simulink library "filteredPID_ul"  (R2022a)
settings: Solver=VariableStepAuto  StartTime=0.0  StopTime=10.0  RelTol=1e-3
settings Model: Creator=adabney  LastModifiedBy=adabney

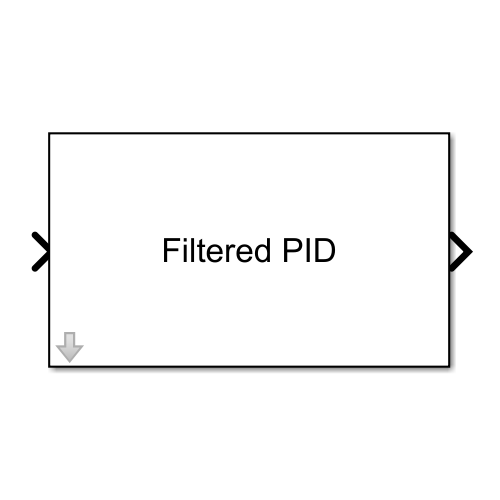
[thumbnail: Simulink's stored preview of the top-level diagram]
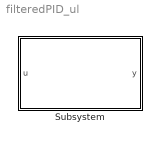
== system filteredPID_ul ==
  Subsystem : Subsystem  mask{kp=0, ki=0, kd=0, tau=0}
      mask prompts: kp "Proportional Gain"; ki "Integral Gain"; kd "Derivative Gain"; tau "Filter Time Constant"
      mask DialogControl ParameterGroupVar Prompt: Control Gains
      mask Display: disp('Filtered PID');

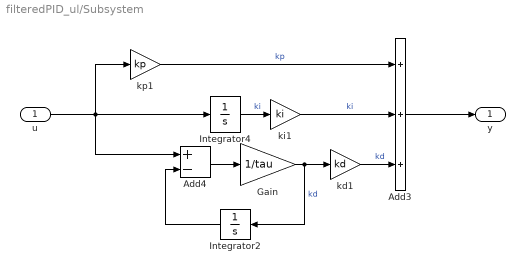
== system filteredPID_ul/Subsystem ==
  u : Inport  PortDimensions=1
  Add3 : Sum  Inputs=+++
  Add4 : Sum  Inputs=+-
  Gain : Gain  Gain=1/tau
  Integrator2 : Integrator  ContinuousStateAttributes='ctrlDerivative'
  Integrator4 : Integrator  ContinuousStateAttributes='ctrlIntegral'
  kd1 : Gain  Gain=kd
  ki1 : Gain  Gain=ki
  kp1 : Gain  Gain=kp
  y : Outport  PortDimensions=1  VectorParamsAs1DForOutWhenUnconnected=off
  wires:
  Add4/1 -> Gain/1
  Integrator2/1 -> Add4/2
  ki1/1 -> Add3/2  "ki"
  kd1/1 -> Add3/3  "kd"
  Integrator4/1 -> ki1/1  "ki"
  u/1 -> Add4/1, kp1/1, Integrator4/1
  Add3/1 -> y/1
  Gain/1 -> Integrator2/1, kd1/1  "kd"
  kp1/1 -> Add3/1  "kp"
